simulink model "lab3_step1"  (R2019b)
settings: Solver=VariableStepAuto  StartTime=0.0  StopTime=5  RelTol=1e-3
InitFcn:
  | W_bits = 32;
  | F_bits = 16;
  | 
  | p = 1;
  | q = 1;
  | 
  | filename ='C:\Users\Louis\Desktop\SoC-FPGAs-II\Lab 3\green_day.wav';
  | 
  | [y,Fs] = audioread(filename);
  | 
  | input_signal = resample(y,p,q);
  | 
  | t = zeros(length(input_signal),1);
  | 
  | for i = 1:length(input_signal)
  |  t(i) = 1/Fs * i*q;
  | end
  | 
  | input_signal = [t input_signal];
StopFcn:
  | output_signal = [out.tout out.output_signal];
  | 
  | sound(output_signal,Fs);
undefined symbols (not defined in the file): Fs
settings Model: Creator=Louis  LastModifiedBy=Louis

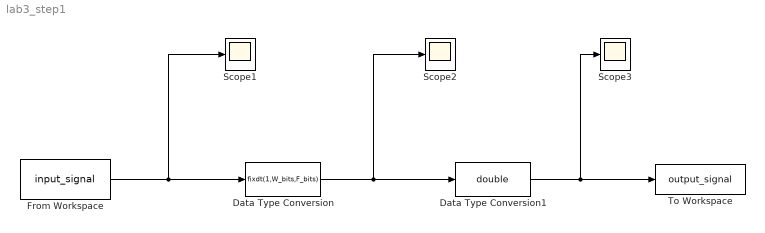
== system lab3_step1 ==
  Data Type Conversion : DataTypeConversion  OutDataTypeStr=fixdt(1,W_bits,F_bits)
  Data Type Conversion1 : DataTypeConversion  OutDataTypeStr=double
  From Workspace : FromWorkspace  VariableName=input_signal  OutDataTypeStr=double  SampleTime=1/Fs*q*4
  Scope1 : Scope
  Scope2 : Scope
  Scope3 : Scope
  To Workspace : ToWorkspace  VariableName=output_signal  SampleTime=1/Fs
      settings: Save2DSignal=2-D array (concatenate along first dimension)
  wires:
  From Workspace/1 -> Data Type Conversion/1, Scope1/1
  Data Type Conversion/1 -> Data Type Conversion1/1, Scope2/1
  Data Type Conversion1/1 -> Scope3/1, To Workspace/1
